simulink model "pendulo2"  (R2017a)
settings: Solver=FixedStepAuto  StartTime=0.0  StopTime=10  FixedStep=0.002  RelTol=1e-3
libraries: cstblocks x3
settings Model: Creator=root  LastModifiedBy=pedro
settings RTWCC: GenCodeOnly=on  PackageGeneratedCodeAndArtifacts=on  PackageName=teste

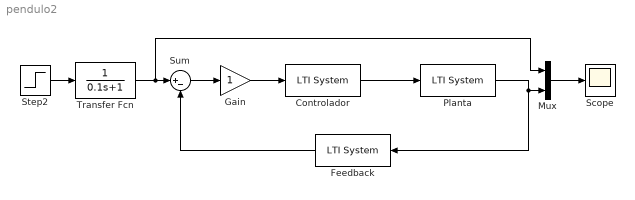
== system pendulo2 ==
  Controlador : cstblocks/LTI System  sys=PID  IC=[]
  Feedback : cstblocks/LTI System  sys=1  IC=[]
  Gain : Gain
  Mux : Mux  Inputs=2
  "Planta " : cstblocks/LTI System  sys=G1  IC=[]
  Scope : Scope
  Step2 : Step  SampleTime=0
  Sum : Sum  Inputs=|+-
  Transfer Fcn : TransferFcn  Denominator=[0.1 1]
  wires:
  Mux/1 -> Scope/1
  Sum/1 -> Gain/1
  Feedback/1 -> Sum/2
  "Planta "/1 -> Feedback/1, Mux/2
  Gain/1 -> Controlador/1
  Controlador/1 -> "Planta "/1
  Transfer Fcn/1 -> Mux/1, Sum/1
  Step2/1 -> Transfer Fcn/1
